simulink library "custom_lib"  (R2021a)
settings: Solver=VariableStepAuto  StartTime=0.0  StopTime=10.0  RelTol=1e-3
libraries: $bdroot x55
settings Model: Creator=Acer  LastModifiedBy=Acer

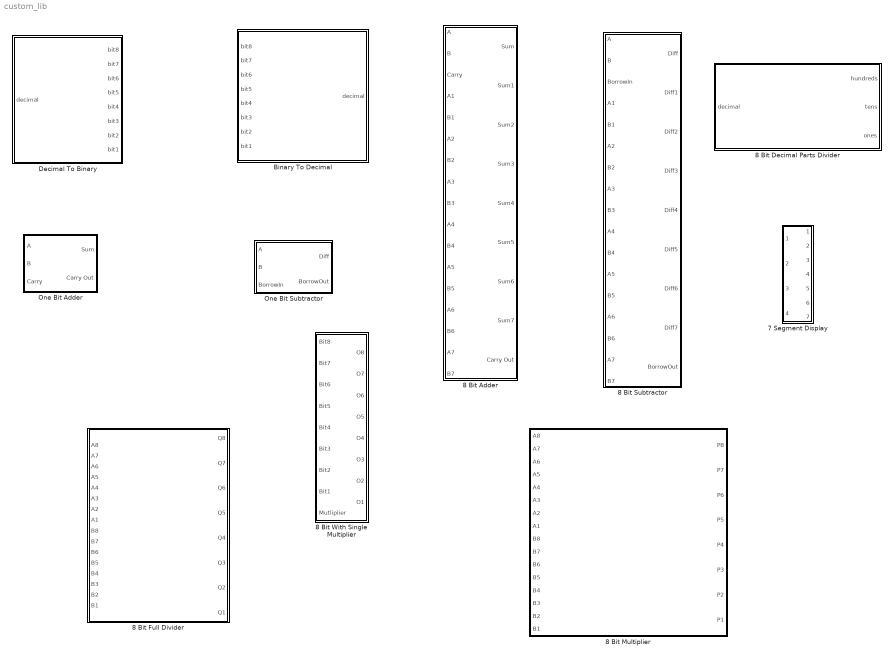
== system custom_lib ==
  7 Segment Display : Subsystem
  8 Bit Adder : Subsystem
  8 Bit Decimal Parts Divider : MATLAB Function  TreatAsAtomicUnit=on
  8 Bit Full Divider : Subsystem
  8 Bit Multiplier : Subsystem
  8 Bit Subtractor : Subsystem
  8 Bit With Single Multiplier : Subsystem
  Binary To Decimal : MATLAB Function  TreatAsAtomicUnit=on
  Decimal To Binary : MATLAB Function  TreatAsAtomicUnit=on
  One Bit Adder : Subsystem
  One Bit Subtractor : Subsystem

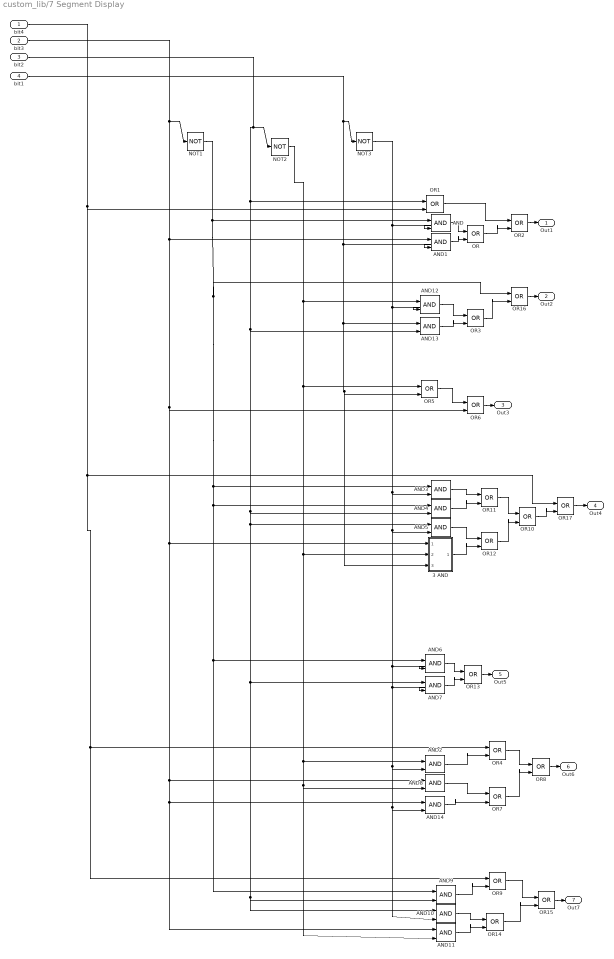
== system custom_lib/7 Segment Display ==
  bit4 : Inport
  bit3 : Inport  Port=2
  bit2 : Inport  Port=3
  bit1 : Inport  Port=4
  3 AND : Subsystem
  AND{,1..14} (15 alike) : Logic  IconShape=distinctive  AllPortsSameDT=off  OutDataTypeStr=boolean
  NOT1 : Logic  Operator=NOT  IconShape=distinctive  AllPortsSameDT=off  OutDataTypeStr=boolean
  NOT2 : Logic  Operator=NOT  IconShape=distinctive  AllPortsSameDT=off  OutDataTypeStr=boolean
  NOT3 : Logic  Operator=NOT  IconShape=distinctive  AllPortsSameDT=off  OutDataTypeStr=boolean
  OR{,1..17} (18 alike) : Logic  Operator=OR  IconShape=distinctive  AllPortsSameDT=off  OutDataTypeStr=boolean
  Out1 : Outport
  Out2 : Outport  Port=2
  Out3 : Outport  Port=3
  Out4 : Outport  Port=4
  Out5 : Outport  Port=5
  Out6 : Outport  Port=6
  Out7 : Outport  Port=7
  wires:
  OR16/1 -> Out2/1
  bit2/1 -> NOT2/1, OR1/1, AND13/2, AND5/1, AND10/1, AND9/2, AND7/1, AND4/2
  NOT2/1 -> OR5/1, AND2/1, AND11/2, AND8/2, 3 AND/2(In2), AND12/1
  bit3/1 -> NOT1/1, AND8/1, AND14/1, AND11/1, 3 AND/1(bit3), OR6/2, AND1/1
  AND7/1 -> OR13/2
  NOT3/1 -> AND/2, AND5/2, AND10/2, AND14/2, AND2/2, AND7/2, AND6/2, AND3/2, AND12/2
  NOT1/1 -> AND/1, OR16/1, AND4/1, AND9/1, AND6/1, AND3/1
  AND9/1 -> OR9/2
  OR3/1 -> OR16/2
  bit4/1 -> OR1/2, OR17/1, OR4/1, OR9/1
  OR4/1 -> OR8/1
  OR7/1 -> OR8/2
  OR17/1 -> Out4/1
  bit1/1 -> AND13/1, 3 AND/3(bit1), OR5/2, AND1/2, NOT3/1
  AND6/1 -> OR13/1
  AND10/1 -> OR14/1
  OR5/1 -> OR6/1
  OR14/1 -> OR15/2
  OR15/1 -> Out7/1
  OR9/1 -> OR15/1
  OR8/1 -> Out6/1
  OR/1 -> OR2/2
  AND2/1 -> OR4/2
  OR13/1 -> Out5/1
  AND8/1 -> OR7/1
  AND11/1 -> OR14/2
  AND12/1 -> OR3/1
  AND14/1 -> OR7/2
  OR1/1 -> OR2/1
  AND/1 -> OR/1
  AND1/1 -> OR/2
  AND13/1 -> OR3/2
  OR6/1 -> Out3/1
  OR2/1 -> Out1/1
  AND3/1 -> OR11/1
  AND4/1 -> OR11/2
  3 AND/1(Out1) -> OR12/2
  AND5/1 -> OR12/1
  OR11/1 -> OR10/1
  OR12/1 -> OR10/2
  OR10/1 -> OR17/2

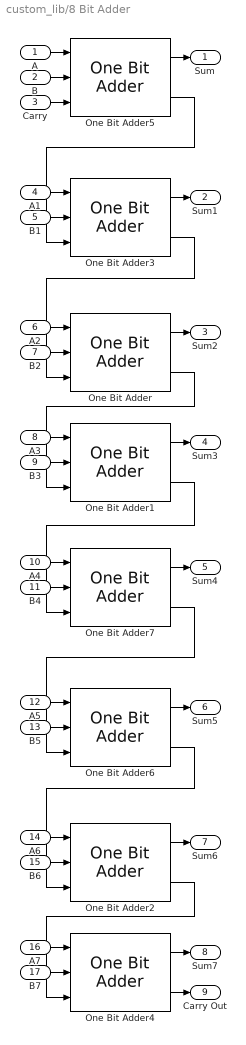
== system custom_lib/8 Bit Adder ==
  A : Inport
  B : Inport  Port=2
  Carry : Inport  Port=3
  A1 : Inport  Port=4
  B1 : Inport  Port=5
  A2 : Inport  Port=6
  B2 : Inport  Port=7
  A3 : Inport  Port=8
  B3 : Inport  Port=9
  A4 : Inport  Port=10
  B4 : Inport  Port=11
  A5 : Inport  Port=12
  B5 : Inport  Port=13
  A6 : Inport  Port=14
  B6 : Inport  Port=15
  A7 : Inport  Port=16
  B7 : Inport  Port=17
  One Bit Adder{,1..7} (8 alike) : $bdroot/One Bit Adder  SystemSampleTime=-1  VariantActivationTime=update diagram  Latency=0  AutoFrameSizeCalculation=off
  Sum : Outport
  Sum1 : Outport  Port=2
  Sum2 : Outport  Port=3
  Sum3 : Outport  Port=4
  Sum4 : Outport  Port=5
  Sum5 : Outport  Port=6
  Sum6 : Outport  Port=7
  Sum7 : Outport  Port=8
  Carry Out : Outport  Port=9
  wires:
  One Bit Adder2/1 -> Sum6/1
  One Bit Adder6/2 -> One Bit Adder2/3
  A1/1 -> One Bit Adder3/1
  One Bit Adder5/2 -> One Bit Adder3/3
  One Bit Adder3/1 -> Sum1/1
  A3/1 -> One Bit Adder1/1
  One Bit Adder7/2 -> One Bit Adder6/3
  One Bit Adder4/2 -> Carry Out/1
  One Bit Adder2/2 -> One Bit Adder4/3
  One Bit Adder3/2 -> One Bit Adder/3
  One Bit Adder/2 -> One Bit Adder1/3
  One Bit Adder1/2 -> One Bit Adder7/3
  One Bit Adder4/1 -> Sum7/1
  One Bit Adder1/1 -> Sum3/1
  B7/1 -> One Bit Adder4/2
  B5/1 -> One Bit Adder6/2
  B/1 -> One Bit Adder5/2
  B2/1 -> One Bit Adder/2
  B6/1 -> One Bit Adder2/2
  A4/1 -> One Bit Adder7/1
  B3/1 -> One Bit Adder1/2
  A2/1 -> One Bit Adder/1
  One Bit Adder/1 -> Sum2/1
  B1/1 -> One Bit Adder3/2
  A6/1 -> One Bit Adder2/1
  A5/1 -> One Bit Adder6/1
  One Bit Adder7/1 -> Sum4/1
  One Bit Adder5/1 -> Sum/1
  One Bit Adder6/1 -> Sum5/1
  B4/1 -> One Bit Adder7/2
  A7/1 -> One Bit Adder4/1
  A/1 -> One Bit Adder5/1
  Carry/1 -> One Bit Adder5/3

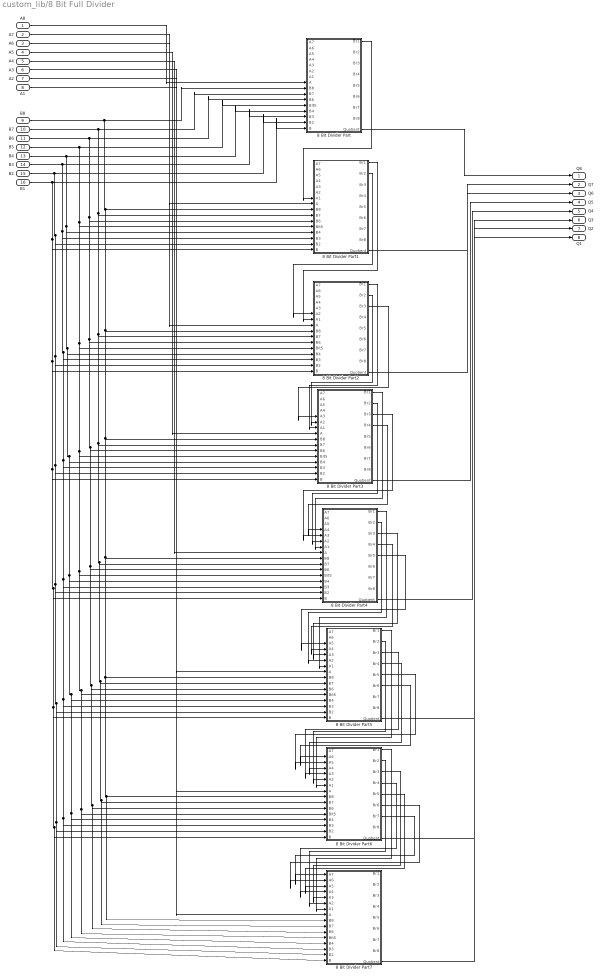
== system custom_lib/8 Bit Full Divider ==
  A8 : Inport
  A7 : Inport  Port=2
  A6 : Inport  Port=3
  A5 : Inport  Port=4
  A4 : Inport  Port=5
  A3 : Inport  Port=6
  A2 : Inport  Port=7
  A1 : Inport  Port=8
  B8 : Inport  Port=9
  B7 : Inport  Port=10
  B6 : Inport  Port=11
  B5 : Inport  Port=12
  B4 : Inport  Port=13
  B3 : Inport  Port=14
  B2 : Inport  Port=15
  B1 : Inport  Port=16
  8 Bit Divider Part : Subsystem
  8 Bit Divider Part1 : Subsystem
  8 Bit Divider Part2 : Subsystem
  8 Bit Divider Part3 : Subsystem
  8 Bit Divider Part4 : Subsystem
  8 Bit Divider Part5 : Subsystem
  8 Bit Divider Part6 : Subsystem
  8 Bit Divider Part7 : Subsystem
  Q8 : Outport
  Q7 : Outport  Port=2
  Q6 : Outport  Port=3
  Q5 : Outport  Port=4
  Q4 : Outport  Port=5
  Q3 : Outport  Port=6
  Q2 : Outport  Port=7
  Q1 : Outport  Port=8
  wires:
  B3/1 -> 8 Bit Divider Part7/14(B3), 8 Bit Divider Part6/14(B3), 8 Bit Divider Part5/14(B3), 8 Bit Divider Part4/14(B3), 8 Bit Divider Part3/14(B3), 8 Bit Divider Part2/14(B3), 8 Bit Divider Part1/14(B3), 8 Bit Divider Part/14(B3)
  B4/1 -> 8 Bit Divider Part7/13(B4), 8 Bit Divider Part6/13(B4), 8 Bit Divider Part5/13(B4), 8 Bit Divider Part4/13(B4), 8 Bit Divider Part3/13(B4), 8 Bit Divider Part2/13(B4), 8 Bit Divider Part1/13(B4), 8 Bit Divider Part/13(B4)
  8 Bit Divider Part2/1(Br1) -> 8 Bit Divider Part3/7(A1)
  8 Bit Divider Part4/1(Br1) -> 8 Bit Divider Part5/7(A1)
  B1/1 -> 8 Bit Divider Part7/16(B), 8 Bit Divider Part6/16(B), 8 Bit Divider Part5/16(B), 8 Bit Divider Part4/16(B), 8 Bit Divider Part3/16(B), 8 Bit Divider Part2/16(B), 8 Bit Divider Part1/16(B), 8 Bit Divider Part/16(B)
  8 Bit Divider Part4/5(Br5) -> 8 Bit Divider Part5/3(A5)
  8 Bit Divider Part6/5(Br5) -> 8 Bit Divider Part7/3(A5)
  A8/1 -> 8 Bit Divider Part/8(A)
  8 Bit Divider Part3/4(Br4) -> 8 Bit Divider Part4/4(A4)
  B2/1 -> 8 Bit Divider Part7/15(B2), 8 Bit Divider Part6/15(B2), 8 Bit Divider Part5/15(B2), 8 Bit Divider Part4/15(B2), 8 Bit Divider Part3/15(B2), 8 Bit Divider Part2/15(B2), 8 Bit Divider Part1/15(B2), 8 Bit Divider Part/15(B2)
  B8/1 -> 8 Bit Divider Part7/9(B8), 8 Bit Divider Part6/9(B8), 8 Bit Divider Part5/9(B8), 8 Bit Divider Part4/9(B8), 8 Bit Divider Part3/9(B8), 8 Bit Divider Part2/9(B8), 8 Bit Divider Part1/9(B8), 8 Bit Divider Part/9(B8)
  B7/1 -> 8 Bit Divider Part7/10(B7), 8 Bit Divider Part6/10(B7), 8 Bit Divider Part5/10(B7), 8 Bit Divider Part4/10(B7), 8 Bit Divider Part3/10(B7), 8 Bit Divider Part2/10(B7), 8 Bit Divider Part1/10(B7), 8 Bit Divider Part/10(B7)
  B6/1 -> 8 Bit Divider Part7/11(B6), 8 Bit Divider Part6/11(B6), 8 Bit Divider Part5/11(B6), 8 Bit Divider Part4/11(B6), 8 Bit Divider Part3/11(B6), 8 Bit Divider Part2/11(B6), 8 Bit Divider Part1/11(B6), 8 Bit Divider Part/11(B6)
  8 Bit Divider Part6/1(Br1) -> 8 Bit Divider Part7/7(A1)
  8 Bit Divider Part2/3(Br3) -> 8 Bit Divider Part3/5(A3)
  8 Bit Divider Part4/2(Br2) -> 8 Bit Divider Part5/6(A2)
  B5/1 -> 8 Bit Divider Part7/12(Bit5), 8 Bit Divider Part6/12(Bit5), 8 Bit Divider Part5/12(Bit5), 8 Bit Divider Part4/12(Bit5), 8 Bit Divider Part3/12(Bit5), 8 Bit Divider Part2/12(Bit5), 8 Bit Divider Part1/12(Bit5), 8 Bit Divider Part/12(Bit5)
  8 Bit Divider Part5/3(Br3) -> 8 Bit Divider Part6/5(A3)
  8 Bit Divider Part3/3(Br3) -> 8 Bit Divider Part4/5(A3)
  8 Bit Divider Part4/3(Br3) -> 8 Bit Divider Part5/5(A3)
  8 Bit Divider Part3/1(Br1) -> 8 Bit Divider Part4/7(A1)
  8 Bit Divider Part5/1(Br1) -> 8 Bit Divider Part6/7(A1)
  8 Bit Divider Part1/1(Br1) -> 8 Bit Divider Part2/7(A1)
  8 Bit Divider Part/1(Br1) -> 8 Bit Divider Part1/7(A1)
  8 Bit Divider Part1/2(Br2) -> 8 Bit Divider Part2/6(A2)
  8 Bit Divider Part6/2(Br2) -> 8 Bit Divider Part7/6(A2)
  A2/1 -> 8 Bit Divider Part6/8(A)
  8 Bit Divider Part2/2(Br2) -> 8 Bit Divider Part3/6(A2)
  8 Bit Divider Part6/4(Br4) -> 8 Bit Divider Part7/4(A4)
  8 Bit Divider Part6/3(Br3) -> 8 Bit Divider Part7/5(A3)
  8 Bit Divider Part5/4(Br4) -> 8 Bit Divider Part6/4(A4)
  8 Bit Divider Part3/2(Br2) -> 8 Bit Divider Part4/6(A2)
  8 Bit Divider Part5/6(Br6) -> 8 Bit Divider Part6/2(A6)
  8 Bit Divider Part4/4(Br4) -> 8 Bit Divider Part5/4(A4)
  8 Bit Divider Part6/6(Br6) -> 8 Bit Divider Part7/2(A6)
  A5/1 -> 8 Bit Divider Part3/8(A)
  8 Bit Divider Part5/2(Br2) -> 8 Bit Divider Part6/6(A2)
  8 Bit Divider Part1/9(Quotient) -> Q7/1
  8 Bit Divider Part2/9(Quotient) -> Q6/1
  8 Bit Divider Part5/5(Br5) -> 8 Bit Divider Part6/3(A5)
  8 Bit Divider Part6/7(Br7) -> 8 Bit Divider Part7/1(A7)
  8 Bit Divider Part/9(Quotient) -> Q8/1
  A6/1 -> 8 Bit Divider Part2/8(A)
  A7/1 -> 8 Bit Divider Part1/8(A)
  A1/1 -> 8 Bit Divider Part7/8(A)
  A4/1 -> 8 Bit Divider Part4/8(A)
  8 Bit Divider Part6/9(Quotient) -> Q2/1
  8 Bit Divider Part5/9(Quotient) -> Q3/1
  A3/1 -> 8 Bit Divider Part5/8(A)
  8 Bit Divider Part3/9(Quotient) -> Q5/1
  8 Bit Divider Part4/9(Quotient) -> Q4/1
  8 Bit Divider Part7/9(Quotient) -> Q1/1

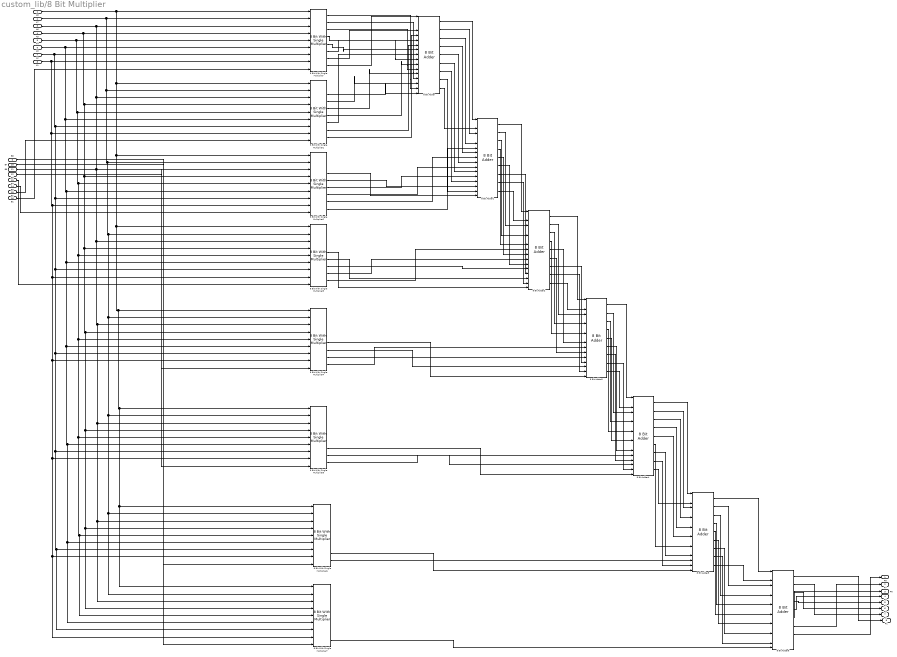
== system custom_lib/8 Bit Multiplier ==
  A8 : Inport
  A7 : Inport  Port=2
  A6 : Inport  Port=3
  A5 : Inport  Port=4
  A4 : Inport  Port=5
  A3 : Inport  Port=6
  A2 : Inport  Port=7
  A1 : Inport  Port=8
  B8 : Inport  Port=9
  B7 : Inport  Port=10
  B6 : Inport  Port=11
  B5 : Inport  Port=12
  B4 : Inport  Port=13
  B3 : Inport  Port=14
  B2 : Inport  Port=15
  B1 : Inport  Port=16
  8 Bit Adder{,1..6} (7 alike) : $bdroot/8 Bit Adder  SystemSampleTime=-1  VariantActivationTime=update diagram  Latency=0  AutoFrameSizeCalculation=off
  8 Bit With Single Multiplier{,1..7} (8 alike) : $bdroot/8 Bit With Single Multiplier  SystemSampleTime=-1  VariantActivationTime=update diagram  Latency=0  AutoFrameSizeCalculation=off
  P8 : Outport
  P7 : Outport  Port=2
  P6 : Outport  Port=3
  P5 : Outport  Port=4
  P4 : Outport  Port=5
  P3 : Outport  Port=6
  P2 : Outport  Port=7
  P1 : Outport  Port=8
  wires:
  8 Bit With Single Multiplier2/5 -> 8 Bit Adder1/13
  A5/1 -> 8 Bit With Single Multiplier7/4, 8 Bit With Single Multiplier6/4, 8 Bit With Single Multiplier5/4, 8 Bit With Single Multiplier4/4, 8 Bit With Single Multiplier3/4, 8 Bit With Single Multiplier2/4, 8 Bit With Single Multiplier1/4, 8 Bit With Single Multiplier/4
  A1/1 -> 8 Bit With Single Multiplier7/8, 8 Bit With Single Multiplier6/8, 8 Bit With Single Multiplier5/8, 8 Bit With Single Multiplier4/8, 8 Bit With Single Multiplier3/8, 8 Bit With Single Multiplier2/8, 8 Bit With Single Multiplier1/8, 8 Bit With Single Multiplier/8
  8 Bit With Single Multiplier3/4 -> 8 Bit Adder2/17
  8 Bit With Single Multiplier5/7 -> 8 Bit Adder4/15
  A2/1 -> 8 Bit With Single Multiplier7/7, 8 Bit With Single Multiplier6/7, 8 Bit With Single Multiplier5/7, 8 Bit With Single Multiplier4/7, 8 Bit With Single Multiplier3/7, 8 Bit With Single Multiplier2/7, 8 Bit With Single Multiplier1/7, 8 Bit With Single Multiplier/7
  8 Bit With Single Multiplier/1 -> 8 Bit Adder/16
  8 Bit With Single Multiplier/2 -> 8 Bit Adder/14
  8 Bit Adder5/2 -> 8 Bit Adder6/4
  8 Bit Adder6/5 -> P5/1
  8 Bit Adder1/4 -> 8 Bit Adder2/8
  8 Bit With Single Multiplier7/8 -> 8 Bit Adder6/17
  8 Bit With Single Multiplier5/6 -> 8 Bit Adder4/17
  8 Bit Adder4/3 -> 8 Bit Adder5/6
  8 Bit Adder3/2 -> 8 Bit Adder4/4
  8 Bit Adder4/2 -> 8 Bit Adder5/4
  8 Bit Adder/2 -> 8 Bit Adder1/4
  8 Bit With Single Multiplier/3 -> 8 Bit Adder/12
  8 Bit Adder5/1 -> 8 Bit Adder6/1
  8 Bit Adder2/4 -> 8 Bit Adder3/8
  8 Bit With Single Multiplier/4 -> 8 Bit Adder/10
  8 Bit Adder4/9 -> 8 Bit Adder5/3
  8 Bit Adder1/9 -> 8 Bit Adder2/3
  8 Bit Adder2/1 -> 8 Bit Adder3/1
  8 Bit With Single Multiplier3/5 -> 8 Bit Adder2/15
  8 Bit Adder5/7 -> 8 Bit Adder6/14
  A8/1 -> 8 Bit With Single Multiplier7/1, 8 Bit With Single Multiplier6/1, 8 Bit With Single Multiplier5/1, 8 Bit With Single Multiplier4/1, 8 Bit With Single Multiplier3/1, 8 Bit With Single Multiplier2/1, 8 Bit With Single Multiplier1/1, 8 Bit With Single Multiplier/1
  8 Bit Adder1/6 -> 8 Bit Adder2/12
  8 Bit Adder5/5 -> 8 Bit Adder6/10
  8 Bit With Single Multiplier2/4 -> 8 Bit Adder1/15
  8 Bit With Single Multiplier/8 -> 8 Bit Adder/1
  8 Bit With Single Multiplier2/7 -> 8 Bit Adder1/9
  8 Bit Adder6/3 -> P3/1
  8 Bit With Single Multiplier1/2 -> 8 Bit Adder/17
  A7/1 -> 8 Bit With Single Multiplier7/2, 8 Bit With Single Multiplier6/2, 8 Bit With Single Multiplier5/2, 8 Bit With Single Multiplier4/2, 8 Bit With Single Multiplier3/2, 8 Bit With Single Multiplier2/2, 8 Bit With Single Multiplier1/2, 8 Bit With Single Multiplier/2
  8 Bit Adder6/2 -> P2/1
  8 Bit With Single Multiplier1/4 -> 8 Bit Adder/13
  8 Bit Adder/1 -> 8 Bit Adder1/1
  A6/1 -> 8 Bit With Single Multiplier7/3, 8 Bit With Single Multiplier6/3, 8 Bit With Single Multiplier5/3, 8 Bit With Single Multiplier4/3, 8 Bit With Single Multiplier3/3, 8 Bit With Single Multiplier2/3, 8 Bit With Single Multiplier1/3, 8 Bit With Single Multiplier/3
  8 Bit Adder/6 -> 8 Bit Adder1/12
  8 Bit Adder1/7 -> 8 Bit Adder2/14
  8 Bit Adder/7 -> 8 Bit Adder1/14
  8 Bit Adder1/8 -> 8 Bit Adder2/16
  A3/1 -> 8 Bit With Single Multiplier7/6, 8 Bit With Single Multiplier6/6, 8 Bit With Single Multiplier5/6, 8 Bit With Single Multiplier4/6, 8 Bit With Single Multiplier3/6, 8 Bit With Single Multiplier2/6, 8 Bit With Single Multiplier1/6, 8 Bit With Single Multiplier/6
  8 Bit With Single Multiplier3/6 -> 8 Bit Adder2/13
  8 Bit With Single Multiplier1/7 -> 8 Bit Adder/7
  8 Bit With Single Multiplier2/8 -> 8 Bit Adder1/7
  8 Bit Adder/3 -> 8 Bit Adder1/6
  8 Bit Adder/5 -> 8 Bit Adder1/10
  8 Bit Adder3/1 -> 8 Bit Adder4/1
  8 Bit Adder1/3 -> 8 Bit Adder2/6
  8 Bit With Single Multiplier1/5 -> 8 Bit Adder/11
  B2/1 -> 8 Bit With Single Multiplier1/9
  8 Bit Adder1/2 -> 8 Bit Adder2/4
  8 Bit Adder/4 -> 8 Bit Adder1/8
  B3/1 -> 8 Bit With Single Multiplier2/9
  8 Bit Adder5/6 -> 8 Bit Adder6/12
  8 Bit Adder1/1 -> 8 Bit Adder2/1
  A4/1 -> 8 Bit With Single Multiplier7/5, 8 Bit With Single Multiplier6/5, 8 Bit With Single Multiplier5/5, 8 Bit With Single Multiplier4/5, 8 Bit With Single Multiplier3/5, 8 Bit With Single Multiplier2/5, 8 Bit With Single Multiplier1/5, 8 Bit With Single Multiplier/5
  8 Bit Adder2/6 -> 8 Bit Adder3/12
  8 Bit Adder2/9 -> 8 Bit Adder3/3
  8 Bit With Single Multiplier1/6 -> 8 Bit Adder/9
  8 Bit Adder3/6 -> 8 Bit Adder4/12
  8 Bit With Single Multiplier/6 -> 8 Bit Adder/6
  8 Bit Adder3/7 -> 8 Bit Adder4/14
  8 Bit Adder2/3 -> 8 Bit Adder3/6
  8 Bit Adder2/5 -> 8 Bit Adder3/10
  8 Bit With Single Multiplier5/8 -> 8 Bit Adder4/13
  8 Bit Adder1/5 -> 8 Bit Adder2/10
  8 Bit Adder2/8 -> 8 Bit Adder3/16
  8 Bit With Single Multiplier3/8 -> 8 Bit Adder2/9
  8 Bit With Single Multiplier4/7 -> 8 Bit Adder3/13
  8 Bit With Single Multiplier/5 -> 8 Bit Adder/8
  8 Bit With Single Multiplier1/3 -> 8 Bit Adder/15
  8 Bit Adder6/4 -> P4/1
  8 Bit Adder3/3 -> 8 Bit Adder4/6
  8 Bit With Single Multiplier4/6 -> 8 Bit Adder3/15
  8 Bit Adder3/9 -> 8 Bit Adder4/3
  8 Bit With Single Multiplier/7 -> 8 Bit Adder/4
  8 Bit Adder3/4 -> 8 Bit Adder4/8
  8 Bit With Single Multiplier6/7 -> 8 Bit Adder5/17
  8 Bit Adder4/4 -> 8 Bit Adder5/8
  8 Bit Adder2/7 -> 8 Bit Adder3/14
  8 Bit With Single Multiplier1/8 -> 8 Bit Adder/5
  8 Bit With Single Multiplier6/8 -> 8 Bit Adder5/15
  8 Bit Adder4/5 -> 8 Bit Adder5/10
  8 Bit With Single Multiplier2/6 -> 8 Bit Adder1/11
  8 Bit Adder4/6 -> 8 Bit Adder5/12
  8 Bit Adder4/1 -> 8 Bit Adder5/1
  8 Bit Adder3/5 -> 8 Bit Adder4/10
  8 Bit Adder2/2 -> 8 Bit Adder3/4
  8 Bit Adder3/8 -> 8 Bit Adder4/16
  8 Bit Adder/8 -> 8 Bit Adder1/16
  8 Bit Adder5/3 -> 8 Bit Adder6/6
  8 Bit Adder5/4 -> 8 Bit Adder6/8
  8 Bit Adder4/8 -> 8 Bit Adder5/16
  8 Bit Adder5/8 -> 8 Bit Adder6/16
  8 Bit With Single Multiplier2/3 -> 8 Bit Adder1/17
  8 Bit Adder4/7 -> 8 Bit Adder5/14
  8 Bit Adder5/9 -> 8 Bit Adder6/3
  8 Bit With Single Multiplier4/5 -> 8 Bit Adder3/17
  8 Bit With Single Multiplier4/8 -> 8 Bit Adder3/11
  8 Bit Adder/9 -> 8 Bit Adder1/3
  8 Bit With Single Multiplier3/7 -> 8 Bit Adder2/11
  8 Bit Adder6/6 -> P6/1
  B5/1 -> 8 Bit With Single Multiplier4/9
  B7/1 -> 8 Bit With Single Multiplier6/9
  B4/1 -> 8 Bit With Single Multiplier3/9
  B8/1 -> 8 Bit With Single Multiplier7/9
  8 Bit Adder6/8 -> P8/1
  B6/1 -> 8 Bit With Single Multiplier5/9
  B1/1 -> 8 Bit With Single Multiplier/9
  8 Bit Adder6/1 -> P1/1
  8 Bit Adder6/7 -> P7/1

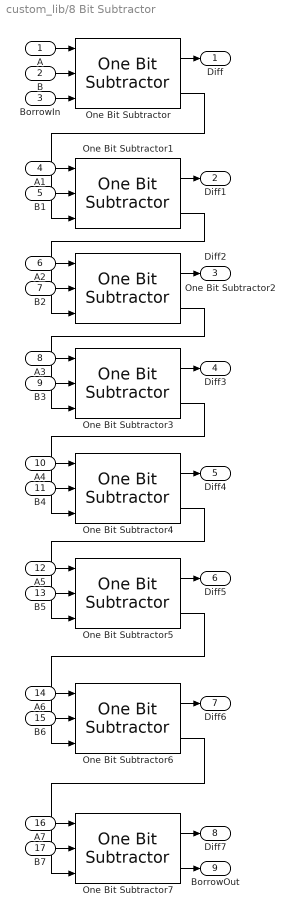
== system custom_lib/8 Bit Subtractor ==
  A : Inport
  B : Inport  Port=2
  BorrowIn : Inport  Port=3
  A1 : Inport  Port=4
  B1 : Inport  Port=5
  A2 : Inport  Port=6
  B2 : Inport  Port=7
  A3 : Inport  Port=8
  B3 : Inport  Port=9
  A4 : Inport  Port=10
  B4 : Inport  Port=11
  A5 : Inport  Port=12
  B5 : Inport  Port=13
  A6 : Inport  Port=14
  B6 : Inport  Port=15
  A7 : Inport  Port=16
  B7 : Inport  Port=17
  One Bit Subtractor{,1..7} (8 alike) : $bdroot/One Bit Subtractor  SystemSampleTime=-1  VariantActivationTime=update diagram  Latency=0  AutoFrameSizeCalculation=off
  Diff : Outport
  Diff1 : Outport  Port=2
  Diff2 : Outport  Port=3
  Diff3 : Outport  Port=4
  Diff4 : Outport  Port=5
  Diff5 : Outport  Port=6
  Diff6 : Outport  Port=7
  Diff7 : Outport  Port=8
  BorrowOut : Outport  Port=9
  wires:
  One Bit Subtractor1/2 -> One Bit Subtractor2/3
  B2/1 -> One Bit Subtractor2/2
  One Bit Subtractor2/2 -> One Bit Subtractor3/3
  One Bit Subtractor3/2 -> One Bit Subtractor4/3
  A3/1 -> One Bit Subtractor3/1
  One Bit Subtractor5/2 -> One Bit Subtractor6/3
  One Bit Subtractor/2 -> One Bit Subtractor1/3
  One Bit Subtractor6/2 -> One Bit Subtractor7/3
  B5/1 -> One Bit Subtractor5/2
  One Bit Subtractor4/2 -> One Bit Subtractor5/3
  B1/1 -> One Bit Subtractor1/2
  One Bit Subtractor5/1 -> Diff5/1
  B6/1 -> One Bit Subtractor6/2
  One Bit Subtractor6/1 -> Diff6/1
  BorrowIn/1 -> One Bit Subtractor/3
  One Bit Subtractor3/1 -> Diff3/1
  One Bit Subtractor4/1 -> Diff4/1
  A5/1 -> One Bit Subtractor5/1
  A2/1 -> One Bit Subtractor2/1
  One Bit Subtractor2/1 -> Diff2/1
  B4/1 -> One Bit Subtractor4/2
  A6/1 -> One Bit Subtractor6/1
  A4/1 -> One Bit Subtractor4/1
  One Bit Subtractor7/1 -> Diff7/1
  B/1 -> One Bit Subtractor/2
  One Bit Subtractor1/1 -> Diff1/1
  A7/1 -> One Bit Subtractor7/1
  A1/1 -> One Bit Subtractor1/1
  A/1 -> One Bit Subtractor/1
  One Bit Subtractor/1 -> Diff/1
  B3/1 -> One Bit Subtractor3/2
  B7/1 -> One Bit Subtractor7/2
  One Bit Subtractor7/2 -> BorrowOut/1

== system custom_lib/8 Bit With Single Multiplier ==
  Bit8 : Inport
  Bit7 : Inport  Port=2
  Bit6 : Inport  Port=3
  Bit5 : Inport  Port=4
  Bit4 : Inport  Port=5
  Bit3 : Inport  Port=6
  Bit2 : Inport  Port=7
  Bit1 : Inport  Port=8
  Mutliplier : Inport  Port=9
  AND{,1..7} (8 alike) : Logic  IconShape=distinctive  AllPortsSameDT=off  OutDataTypeStr=boolean
  O8 : Outport
  O7 : Outport  Port=2
  O6 : Outport  Port=3
  O5 : Outport  Port=4
  O4 : Outport  Port=5
  O3 : Outport  Port=6
  O2 : Outport  Port=7
  O1 : Outport  Port=8
  wires:
  Mutliplier/1 -> AND/2, AND1/2, AND2/2, AND3/2, AND6/2, AND7/2, AND5/2, AND4/2
  AND/1 -> O8/1
  AND3/1 -> O5/1
  Bit8/1 -> AND/1
  Bit5/1 -> AND3/1
  AND2/1 -> O6/1
  AND5/1 -> O2/1
  AND7/1 -> O3/1
  Bit3/1 -> AND7/1
  Bit1/1 -> AND4/1
  Bit4/1 -> AND6/1
  AND6/1 -> O4/1
  Bit7/1 -> AND1/1
  Bit2/1 -> AND5/1
  AND1/1 -> O7/1
  Bit6/1 -> AND2/1
  AND4/1 -> O1/1

== system custom_lib/One Bit Adder ==
  A : Inport
  B : Inport  Port=2
  Carry : Inport  Port=3
  AND : Logic  IconShape=distinctive  AllPortsSameDT=off  OutDataTypeStr=boolean
  AND1 : Logic  IconShape=distinctive  AllPortsSameDT=off  OutDataTypeStr=boolean
  OR : Logic  Operator=OR  IconShape=distinctive  AllPortsSameDT=off  OutDataTypeStr=boolean
  XOR : Logic  Operator=XOR  IconShape=distinctive  AllPortsSameDT=off  OutDataTypeStr=boolean
  XOR1 : Logic  Operator=XOR  IconShape=distinctive  AllPortsSameDT=off  OutDataTypeStr=boolean
  Sum : Outport
  Carry Out : Outport  Port=2
  wires:
  AND1/1 -> OR/2
  XOR1/1 -> Sum/1
  Carry/1 -> XOR1/2, AND/2
  B/1 -> AND1/2, XOR/2
  A/1 -> AND1/1, XOR/1
  OR/1 -> Carry Out/1
  AND/1 -> OR/1
  XOR/1 -> AND/1, XOR1/1

== system custom_lib/One Bit Subtractor ==
  A : Inport
  B : Inport  Port=2
  BorrowIn : Inport  Port=3
  AND : Logic  IconShape=distinctive  AllPortsSameDT=off  OutDataTypeStr=boolean
  AND1 : Logic  IconShape=distinctive  AllPortsSameDT=off  OutDataTypeStr=boolean
  NOT : Logic  Operator=NOT  IconShape=distinctive  AllPortsSameDT=off  OutDataTypeStr=boolean
  NOT1 : Logic  Operator=NOT  IconShape=distinctive  AllPortsSameDT=off  OutDataTypeStr=boolean
  OR : Logic  Operator=OR  IconShape=distinctive  AllPortsSameDT=off  OutDataTypeStr=boolean
  XOR : Logic  Operator=XOR  IconShape=distinctive  AllPortsSameDT=off  OutDataTypeStr=boolean
  XOR1 : Logic  Operator=XOR  IconShape=distinctive  AllPortsSameDT=off  OutDataTypeStr=boolean
  Diff : Outport
  BorrowOut : Outport  Port=2
  wires:
  BorrowIn/1 -> AND1/2, XOR1/2
  AND/1 -> OR/2
  A/1 -> NOT/1, XOR/1
  B/1 -> AND/2, XOR/2
  XOR/1 -> NOT1/1, XOR1/1
  NOT1/1 -> AND1/1
  XOR1/1 -> Diff/1
  NOT/1 -> AND/1
  AND1/1 -> OR/1
  OR/1 -> BorrowOut/1

== system custom_lib/7 Segment Display/3 AND ==
  bit3 : Inport
  In2 : Inport  Port=2
  bit1 : Inport  Port=3
  AND15 : Logic  IconShape=distinctive  AllPortsSameDT=off  OutDataTypeStr=boolean
  AND16 : Logic  IconShape=distinctive  AllPortsSameDT=off  OutDataTypeStr=boolean
  Out1 : Outport
  wires:
  In2/1 -> AND15/2
  AND16/1 -> Out1/1
  AND15/1 -> AND16/1
  bit3/1 -> AND15/1
  bit1/1 -> AND16/2

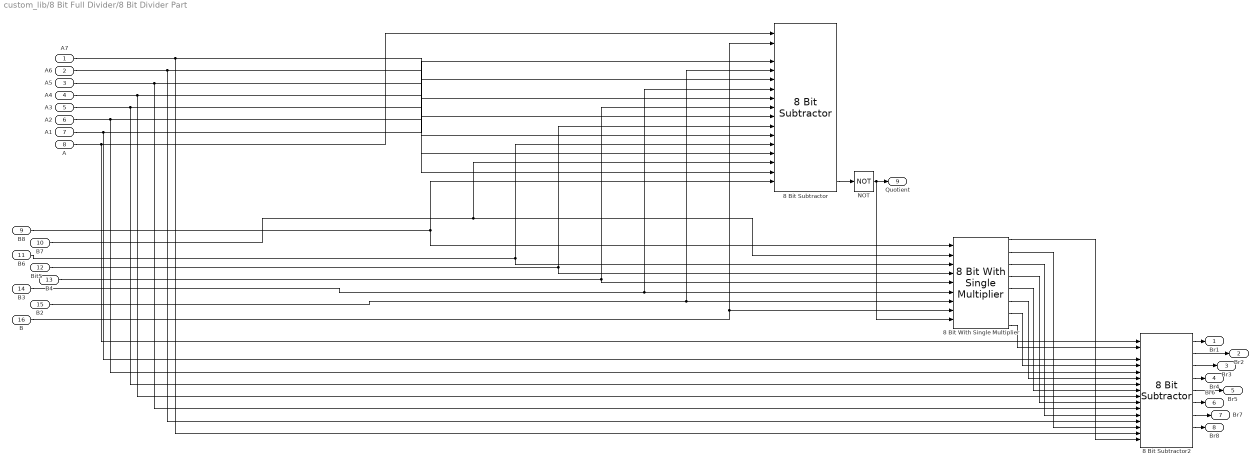
== system custom_lib/8 Bit Full Divider/8 Bit Divider Part ==
  A7 : Inport
  A6 : Inport  Port=2
  A5 : Inport  Port=3
  A4 : Inport  Port=4
  A3 : Inport  Port=5
  A2 : Inport  Port=6
  A1 : Inport  Port=7
  A : Inport  Port=8
  B8 : Inport  Port=9
  B7 : Inport  Port=10
  B6 : Inport  Port=11
  Bit5 : Inport  Port=12
  B4 : Inport  Port=13
  B3 : Inport  Port=14
  B2 : Inport  Port=15
  B : Inport  Port=16
  8 Bit Subtractor : $bdroot/8 Bit Subtractor  SystemSampleTime=-1  VariantActivationTime=update diagram  Latency=0  AutoFrameSizeCalculation=off
  8 Bit Subtractor2 : $bdroot/8 Bit Subtractor  SystemSampleTime=-1  VariantActivationTime=update diagram  Latency=0  AutoFrameSizeCalculation=off
  8 Bit With Single Multiplier : $bdroot/8 Bit With Single Multiplier  SystemSampleTime=-1  VariantActivationTime=update diagram  Latency=0  AutoFrameSizeCalculation=off
  NOT : Logic  Operator=NOT  IconShape=distinctive  AllPortsSameDT=off  OutDataTypeStr=boolean
  Br1 : Outport
  Br2 : Outport  Port=2
  Br3 : Outport  Port=3
  Br4 : Outport  Port=4
  Br5 : Outport  Port=5
  Br6 : Outport  Port=6
  Br7 : Outport  Port=7
  Br8 : Outport  Port=8
  Quotient : Outport  Port=9
  wires:
  8 Bit Subtractor2/3 -> Br3/1
  8 Bit With Single Multiplier/2 -> 8 Bit Subtractor2/15
  8 Bit With Single Multiplier/7 -> 8 Bit Subtractor2/5
  B2/1 -> 8 Bit Subtractor/5, 8 Bit With Single Multiplier/7
  B6/1 -> 8 Bit Subtractor/13, 8 Bit With Single Multiplier/3
  8 Bit With Single Multiplier/1 -> 8 Bit Subtractor2/17
  8 Bit Subtractor2/6 -> Br6/1
  A7/1 -> 8 Bit Subtractor2/16, 8 Bit Subtractor/16
  NOT/1 -> Quotient/1, 8 Bit With Single Multiplier/9
  B8/1 -> 8 Bit Subtractor/17, 8 Bit With Single Multiplier/1
  A/1 -> 8 Bit Subtractor2/1, 8 Bit Subtractor/1
  A3/1 -> 8 Bit Subtractor2/8, 8 Bit Subtractor/8
  8 Bit Subtractor2/8 -> Br8/1
  B4/1 -> 8 Bit Subtractor/9, 8 Bit With Single Multiplier/5
  A2/1 -> 8 Bit Subtractor2/6, 8 Bit Subtractor/6
  8 Bit Subtractor2/2 -> Br2/1
  8 Bit With Single Multiplier/3 -> 8 Bit Subtractor2/13
  B7/1 -> 8 Bit With Single Multiplier/2, 8 Bit Subtractor/15
  8 Bit Subtractor/9 -> NOT/1
  B3/1 -> 8 Bit Subtractor/7, 8 Bit With Single Multiplier/6
  Bit5/1 -> 8 Bit Subtractor/11, 8 Bit With Single Multiplier/4
  8 Bit With Single Multiplier/8 -> 8 Bit Subtractor2/2
  8 Bit With Single Multiplier/5 -> 8 Bit Subtractor2/9
  8 Bit With Single Multiplier/6 -> 8 Bit Subtractor2/7
  8 Bit Subtractor2/4 -> Br4/1
  8 Bit Subtractor2/7 -> Br7/1
  8 Bit With Single Multiplier/4 -> 8 Bit Subtractor2/11
  B/1 -> 8 Bit With Single Multiplier/8, 8 Bit Subtractor/2
  8 Bit Subtractor2/5 -> Br5/1
  A1/1 -> 8 Bit Subtractor2/4, 8 Bit Subtractor/4
  A6/1 -> 8 Bit Subtractor2/14, 8 Bit Subtractor/14
  8 Bit Subtractor2/1 -> Br1/1
  A4/1 -> 8 Bit Subtractor2/10, 8 Bit Subtractor/10
  A5/1 -> 8 Bit Subtractor2/12, 8 Bit Subtractor/12

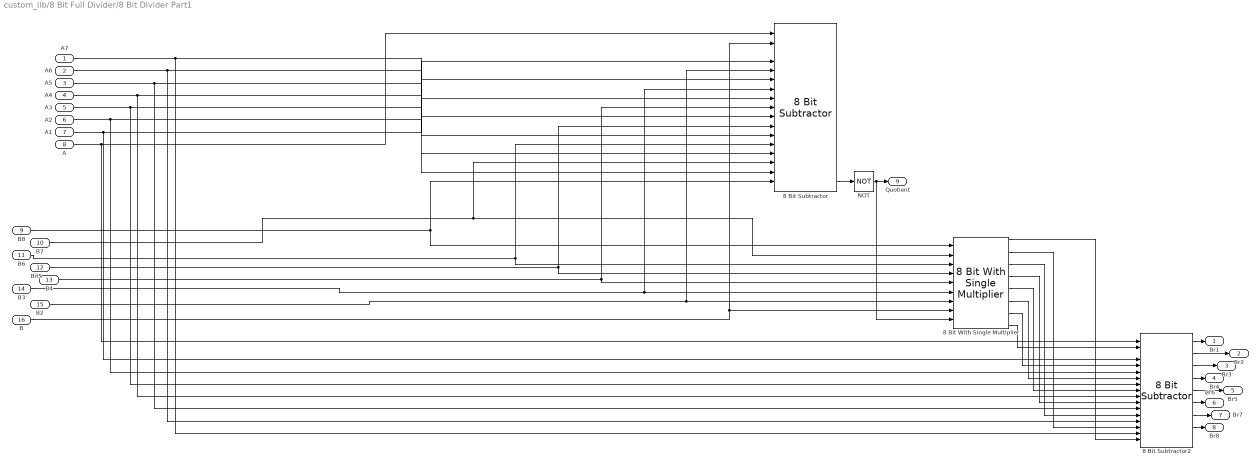
== system custom_lib/8 Bit Full Divider/8 Bit Divider Part1 ==
  A7 : Inport
  A6 : Inport  Port=2
  A5 : Inport  Port=3
  A4 : Inport  Port=4
  A3 : Inport  Port=5
  A2 : Inport  Port=6
  A1 : Inport  Port=7
  A : Inport  Port=8
  B8 : Inport  Port=9
  B7 : Inport  Port=10
  B6 : Inport  Port=11
  Bit5 : Inport  Port=12
  B4 : Inport  Port=13
  B3 : Inport  Port=14
  B2 : Inport  Port=15
  B : Inport  Port=16
  8 Bit Subtractor : $bdroot/8 Bit Subtractor  SystemSampleTime=-1  VariantActivationTime=update diagram  Latency=0  AutoFrameSizeCalculation=off
  8 Bit Subtractor2 : $bdroot/8 Bit Subtractor  SystemSampleTime=-1  VariantActivationTime=update diagram  Latency=0  AutoFrameSizeCalculation=off
  8 Bit With Single Multiplier : $bdroot/8 Bit With Single Multiplier  SystemSampleTime=-1  VariantActivationTime=update diagram  Latency=0  AutoFrameSizeCalculation=off
  NOT : Logic  Operator=NOT  IconShape=distinctive  AllPortsSameDT=off  OutDataTypeStr=boolean
  Br1 : Outport
  Br2 : Outport  Port=2
  Br3 : Outport  Port=3
  Br4 : Outport  Port=4
  Br5 : Outport  Port=5
  Br6 : Outport  Port=6
  Br7 : Outport  Port=7
  Br8 : Outport  Port=8
  Quotient : Outport  Port=9
  wires:
  8 Bit Subtractor2/3 -> Br3/1
  8 Bit With Single Multiplier/2 -> 8 Bit Subtractor2/15
  8 Bit With Single Multiplier/7 -> 8 Bit Subtractor2/5
  B2/1 -> 8 Bit Subtractor/5, 8 Bit With Single Multiplier/7
  B6/1 -> 8 Bit Subtractor/13, 8 Bit With Single Multiplier/3
  8 Bit With Single Multiplier/1 -> 8 Bit Subtractor2/17
  8 Bit Subtractor2/6 -> Br6/1
  A7/1 -> 8 Bit Subtractor2/16, 8 Bit Subtractor/16
  NOT/1 -> Quotient/1, 8 Bit With Single Multiplier/9
  B8/1 -> 8 Bit Subtractor/17, 8 Bit With Single Multiplier/1
  A/1 -> 8 Bit Subtractor2/1, 8 Bit Subtractor/1
  A3/1 -> 8 Bit Subtractor2/8, 8 Bit Subtractor/8
  8 Bit Subtractor2/8 -> Br8/1
  B4/1 -> 8 Bit Subtractor/9, 8 Bit With Single Multiplier/5
  A2/1 -> 8 Bit Subtractor2/6, 8 Bit Subtractor/6
  8 Bit Subtractor2/2 -> Br2/1
  8 Bit With Single Multiplier/3 -> 8 Bit Subtractor2/13
  B7/1 -> 8 Bit With Single Multiplier/2, 8 Bit Subtractor/15
  8 Bit Subtractor/9 -> NOT/1
  B3/1 -> 8 Bit Subtractor/7, 8 Bit With Single Multiplier/6
  Bit5/1 -> 8 Bit Subtractor/11, 8 Bit With Single Multiplier/4
  8 Bit With Single Multiplier/8 -> 8 Bit Subtractor2/2
  8 Bit With Single Multiplier/5 -> 8 Bit Subtractor2/9
  8 Bit With Single Multiplier/6 -> 8 Bit Subtractor2/7
  8 Bit Subtractor2/4 -> Br4/1
  8 Bit Subtractor2/7 -> Br7/1
  8 Bit With Single Multiplier/4 -> 8 Bit Subtractor2/11
  B/1 -> 8 Bit With Single Multiplier/8, 8 Bit Subtractor/2
  8 Bit Subtractor2/5 -> Br5/1
  A1/1 -> 8 Bit Subtractor2/4, 8 Bit Subtractor/4
  A6/1 -> 8 Bit Subtractor2/14, 8 Bit Subtractor/14
  8 Bit Subtractor2/1 -> Br1/1
  A4/1 -> 8 Bit Subtractor2/10, 8 Bit Subtractor/10
  A5/1 -> 8 Bit Subtractor2/12, 8 Bit Subtractor/12

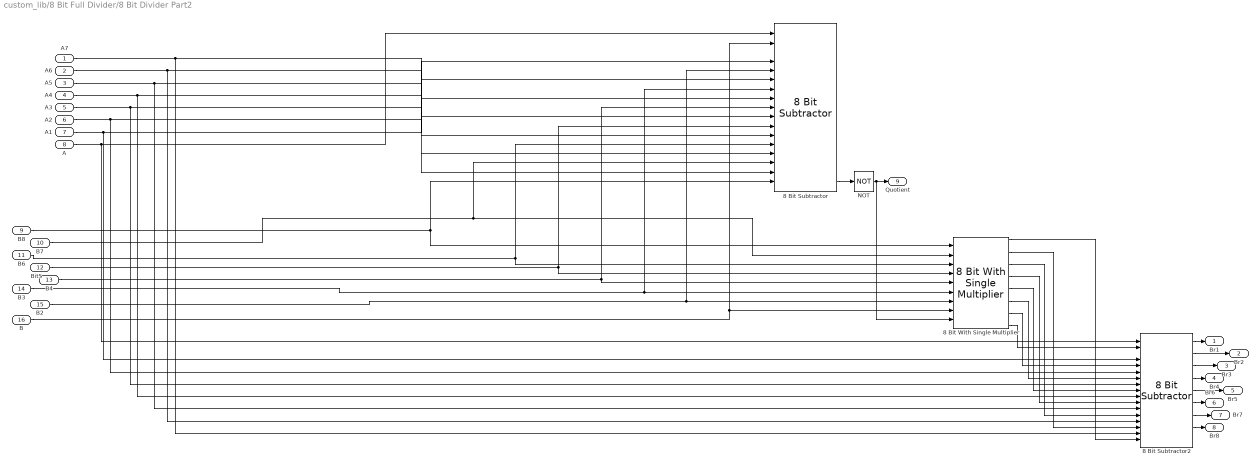
== system custom_lib/8 Bit Full Divider/8 Bit Divider Part2 ==
  A7 : Inport
  A6 : Inport  Port=2
  A5 : Inport  Port=3
  A4 : Inport  Port=4
  A3 : Inport  Port=5
  A2 : Inport  Port=6
  A1 : Inport  Port=7
  A : Inport  Port=8
  B8 : Inport  Port=9
  B7 : Inport  Port=10
  B6 : Inport  Port=11
  Bit5 : Inport  Port=12
  B4 : Inport  Port=13
  B3 : Inport  Port=14
  B2 : Inport  Port=15
  B : Inport  Port=16
  8 Bit Subtractor : $bdroot/8 Bit Subtractor  SystemSampleTime=-1  VariantActivationTime=update diagram  Latency=0  AutoFrameSizeCalculation=off
  8 Bit Subtractor2 : $bdroot/8 Bit Subtractor  SystemSampleTime=-1  VariantActivationTime=update diagram  Latency=0  AutoFrameSizeCalculation=off
  8 Bit With Single Multiplier : $bdroot/8 Bit With Single Multiplier  SystemSampleTime=-1  VariantActivationTime=update diagram  Latency=0  AutoFrameSizeCalculation=off
  NOT : Logic  Operator=NOT  IconShape=distinctive  AllPortsSameDT=off  OutDataTypeStr=boolean
  Br1 : Outport
  Br2 : Outport  Port=2
  Br3 : Outport  Port=3
  Br4 : Outport  Port=4
  Br5 : Outport  Port=5
  Br6 : Outport  Port=6
  Br7 : Outport  Port=7
  Br8 : Outport  Port=8
  Quotient : Outport  Port=9
  wires:
  8 Bit Subtractor2/3 -> Br3/1
  8 Bit With Single Multiplier/2 -> 8 Bit Subtractor2/15
  8 Bit With Single Multiplier/7 -> 8 Bit Subtractor2/5
  B2/1 -> 8 Bit Subtractor/5, 8 Bit With Single Multiplier/7
  B6/1 -> 8 Bit Subtractor/13, 8 Bit With Single Multiplier/3
  8 Bit With Single Multiplier/1 -> 8 Bit Subtractor2/17
  8 Bit Subtractor2/6 -> Br6/1
  A7/1 -> 8 Bit Subtractor2/16, 8 Bit Subtractor/16
  NOT/1 -> Quotient/1, 8 Bit With Single Multiplier/9
  B8/1 -> 8 Bit Subtractor/17, 8 Bit With Single Multiplier/1
  A/1 -> 8 Bit Subtractor2/1, 8 Bit Subtractor/1
  A3/1 -> 8 Bit Subtractor2/8, 8 Bit Subtractor/8
  8 Bit Subtractor2/8 -> Br8/1
  B4/1 -> 8 Bit Subtractor/9, 8 Bit With Single Multiplier/5
  A2/1 -> 8 Bit Subtractor2/6, 8 Bit Subtractor/6
  8 Bit Subtractor2/2 -> Br2/1
  8 Bit With Single Multiplier/3 -> 8 Bit Subtractor2/13
  B7/1 -> 8 Bit With Single Multiplier/2, 8 Bit Subtractor/15
  8 Bit Subtractor/9 -> NOT/1
  B3/1 -> 8 Bit Subtractor/7, 8 Bit With Single Multiplier/6
  Bit5/1 -> 8 Bit Subtractor/11, 8 Bit With Single Multiplier/4
  8 Bit With Single Multiplier/8 -> 8 Bit Subtractor2/2
  8 Bit With Single Multiplier/5 -> 8 Bit Subtractor2/9
  8 Bit With Single Multiplier/6 -> 8 Bit Subtractor2/7
  8 Bit Subtractor2/4 -> Br4/1
  8 Bit Subtractor2/7 -> Br7/1
  8 Bit With Single Multiplier/4 -> 8 Bit Subtractor2/11
  B/1 -> 8 Bit With Single Multiplier/8, 8 Bit Subtractor/2
  8 Bit Subtractor2/5 -> Br5/1
  A1/1 -> 8 Bit Subtractor2/4, 8 Bit Subtractor/4
  A6/1 -> 8 Bit Subtractor2/14, 8 Bit Subtractor/14
  8 Bit Subtractor2/1 -> Br1/1
  A4/1 -> 8 Bit Subtractor2/10, 8 Bit Subtractor/10
  A5/1 -> 8 Bit Subtractor2/12, 8 Bit Subtractor/12

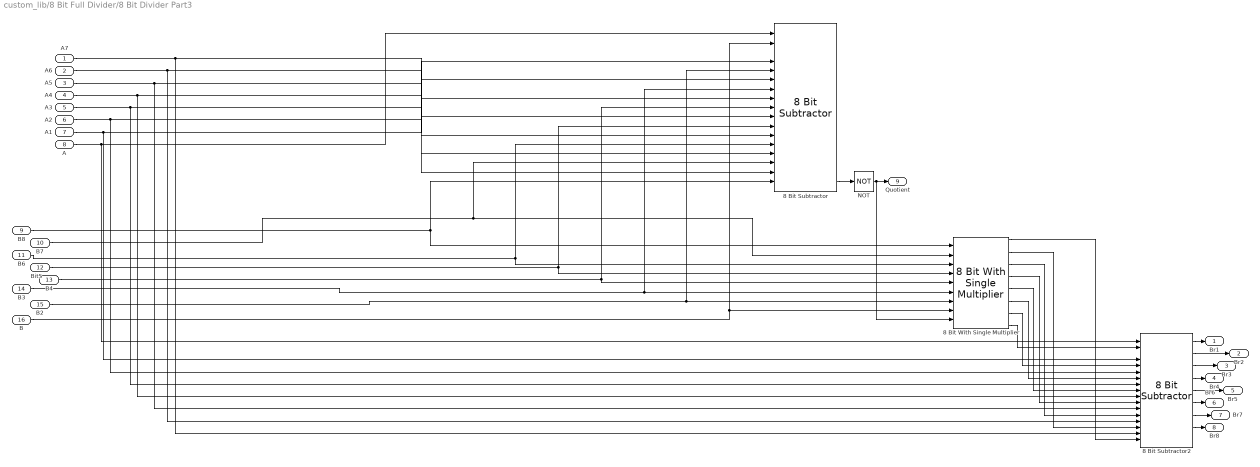
== system custom_lib/8 Bit Full Divider/8 Bit Divider Part3 ==
  A7 : Inport
  A6 : Inport  Port=2
  A5 : Inport  Port=3
  A4 : Inport  Port=4
  A3 : Inport  Port=5
  A2 : Inport  Port=6
  A1 : Inport  Port=7
  A : Inport  Port=8
  B8 : Inport  Port=9
  B7 : Inport  Port=10
  B6 : Inport  Port=11
  Bit5 : Inport  Port=12
  B4 : Inport  Port=13
  B3 : Inport  Port=14
  B2 : Inport  Port=15
  B : Inport  Port=16
  8 Bit Subtractor : $bdroot/8 Bit Subtractor  SystemSampleTime=-1  VariantActivationTime=update diagram  Latency=0  AutoFrameSizeCalculation=off
  8 Bit Subtractor2 : $bdroot/8 Bit Subtractor  SystemSampleTime=-1  VariantActivationTime=update diagram  Latency=0  AutoFrameSizeCalculation=off
  8 Bit With Single Multiplier : $bdroot/8 Bit With Single Multiplier  SystemSampleTime=-1  VariantActivationTime=update diagram  Latency=0  AutoFrameSizeCalculation=off
  NOT : Logic  Operator=NOT  IconShape=distinctive  AllPortsSameDT=off  OutDataTypeStr=boolean
  Br1 : Outport
  Br2 : Outport  Port=2
  Br3 : Outport  Port=3
  Br4 : Outport  Port=4
  Br5 : Outport  Port=5
  Br6 : Outport  Port=6
  Br7 : Outport  Port=7
  Br8 : Outport  Port=8
  Quotient : Outport  Port=9
  wires:
  8 Bit Subtractor2/3 -> Br3/1
  8 Bit With Single Multiplier/2 -> 8 Bit Subtractor2/15
  8 Bit With Single Multiplier/7 -> 8 Bit Subtractor2/5
  B2/1 -> 8 Bit Subtractor/5, 8 Bit With Single Multiplier/7
  B6/1 -> 8 Bit Subtractor/13, 8 Bit With Single Multiplier/3
  8 Bit With Single Multiplier/1 -> 8 Bit Subtractor2/17
  8 Bit Subtractor2/6 -> Br6/1
  A7/1 -> 8 Bit Subtractor2/16, 8 Bit Subtractor/16
  NOT/1 -> Quotient/1, 8 Bit With Single Multiplier/9
  B8/1 -> 8 Bit Subtractor/17, 8 Bit With Single Multiplier/1
  A/1 -> 8 Bit Subtractor2/1, 8 Bit Subtractor/1
  A3/1 -> 8 Bit Subtractor2/8, 8 Bit Subtractor/8
  8 Bit Subtractor2/8 -> Br8/1
  B4/1 -> 8 Bit Subtractor/9, 8 Bit With Single Multiplier/5
  A2/1 -> 8 Bit Subtractor2/6, 8 Bit Subtractor/6
  8 Bit Subtractor2/2 -> Br2/1
  8 Bit With Single Multiplier/3 -> 8 Bit Subtractor2/13
  B7/1 -> 8 Bit With Single Multiplier/2, 8 Bit Subtractor/15
  8 Bit Subtractor/9 -> NOT/1
  B3/1 -> 8 Bit Subtractor/7, 8 Bit With Single Multiplier/6
  Bit5/1 -> 8 Bit Subtractor/11, 8 Bit With Single Multiplier/4
  8 Bit With Single Multiplier/8 -> 8 Bit Subtractor2/2
  8 Bit With Single Multiplier/5 -> 8 Bit Subtractor2/9
  8 Bit With Single Multiplier/6 -> 8 Bit Subtractor2/7
  8 Bit Subtractor2/4 -> Br4/1
  8 Bit Subtractor2/7 -> Br7/1
  8 Bit With Single Multiplier/4 -> 8 Bit Subtractor2/11
  B/1 -> 8 Bit With Single Multiplier/8, 8 Bit Subtractor/2
  8 Bit Subtractor2/5 -> Br5/1
  A1/1 -> 8 Bit Subtractor2/4, 8 Bit Subtractor/4
  A6/1 -> 8 Bit Subtractor2/14, 8 Bit Subtractor/14
  8 Bit Subtractor2/1 -> Br1/1
  A4/1 -> 8 Bit Subtractor2/10, 8 Bit Subtractor/10
  A5/1 -> 8 Bit Subtractor2/12, 8 Bit Subtractor/12

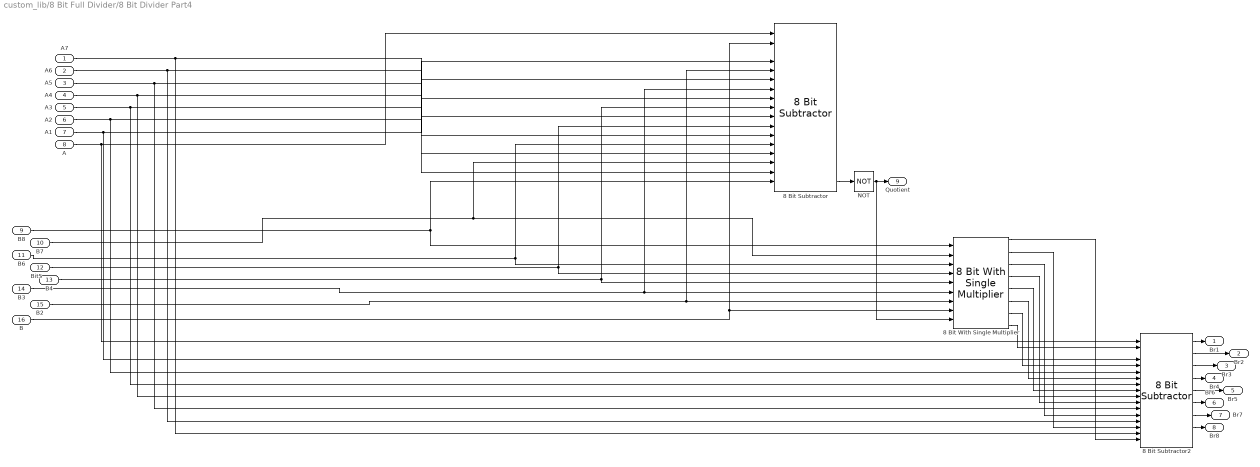
== system custom_lib/8 Bit Full Divider/8 Bit Divider Part4 ==
  A7 : Inport
  A6 : Inport  Port=2
  A5 : Inport  Port=3
  A4 : Inport  Port=4
  A3 : Inport  Port=5
  A2 : Inport  Port=6
  A1 : Inport  Port=7
  A : Inport  Port=8
  B8 : Inport  Port=9
  B7 : Inport  Port=10
  B6 : Inport  Port=11
  Bit5 : Inport  Port=12
  B4 : Inport  Port=13
  B3 : Inport  Port=14
  B2 : Inport  Port=15
  B : Inport  Port=16
  8 Bit Subtractor : $bdroot/8 Bit Subtractor  SystemSampleTime=-1  VariantActivationTime=update diagram  Latency=0  AutoFrameSizeCalculation=off
  8 Bit Subtractor2 : $bdroot/8 Bit Subtractor  SystemSampleTime=-1  VariantActivationTime=update diagram  Latency=0  AutoFrameSizeCalculation=off
  8 Bit With Single Multiplier : $bdroot/8 Bit With Single Multiplier  SystemSampleTime=-1  VariantActivationTime=update diagram  Latency=0  AutoFrameSizeCalculation=off
  NOT : Logic  Operator=NOT  IconShape=distinctive  AllPortsSameDT=off  OutDataTypeStr=boolean
  Br1 : Outport
  Br2 : Outport  Port=2
  Br3 : Outport  Port=3
  Br4 : Outport  Port=4
  Br5 : Outport  Port=5
  Br6 : Outport  Port=6
  Br7 : Outport  Port=7
  Br8 : Outport  Port=8
  Quotient : Outport  Port=9
  wires:
  8 Bit Subtractor2/3 -> Br3/1
  8 Bit With Single Multiplier/2 -> 8 Bit Subtractor2/15
  8 Bit With Single Multiplier/7 -> 8 Bit Subtractor2/5
  B2/1 -> 8 Bit Subtractor/5, 8 Bit With Single Multiplier/7
  B6/1 -> 8 Bit Subtractor/13, 8 Bit With Single Multiplier/3
  8 Bit With Single Multiplier/1 -> 8 Bit Subtractor2/17
  8 Bit Subtractor2/6 -> Br6/1
  A7/1 -> 8 Bit Subtractor2/16, 8 Bit Subtractor/16
  NOT/1 -> Quotient/1, 8 Bit With Single Multiplier/9
  B8/1 -> 8 Bit Subtractor/17, 8 Bit With Single Multiplier/1
  A/1 -> 8 Bit Subtractor2/1, 8 Bit Subtractor/1
  A3/1 -> 8 Bit Subtractor2/8, 8 Bit Subtractor/8
  8 Bit Subtractor2/8 -> Br8/1
  B4/1 -> 8 Bit Subtractor/9, 8 Bit With Single Multiplier/5
  A2/1 -> 8 Bit Subtractor2/6, 8 Bit Subtractor/6
  8 Bit Subtractor2/2 -> Br2/1
  8 Bit With Single Multiplier/3 -> 8 Bit Subtractor2/13
  B7/1 -> 8 Bit With Single Multiplier/2, 8 Bit Subtractor/15
  8 Bit Subtractor/9 -> NOT/1
  B3/1 -> 8 Bit Subtractor/7, 8 Bit With Single Multiplier/6
  Bit5/1 -> 8 Bit Subtractor/11, 8 Bit With Single Multiplier/4
  8 Bit With Single Multiplier/8 -> 8 Bit Subtractor2/2
  8 Bit With Single Multiplier/5 -> 8 Bit Subtractor2/9
  8 Bit With Single Multiplier/6 -> 8 Bit Subtractor2/7
  8 Bit Subtractor2/4 -> Br4/1
  8 Bit Subtractor2/7 -> Br7/1
  8 Bit With Single Multiplier/4 -> 8 Bit Subtractor2/11
  B/1 -> 8 Bit With Single Multiplier/8, 8 Bit Subtractor/2
  8 Bit Subtractor2/5 -> Br5/1
  A1/1 -> 8 Bit Subtractor2/4, 8 Bit Subtractor/4
  A6/1 -> 8 Bit Subtractor2/14, 8 Bit Subtractor/14
  8 Bit Subtractor2/1 -> Br1/1
  A4/1 -> 8 Bit Subtractor2/10, 8 Bit Subtractor/10
  A5/1 -> 8 Bit Subtractor2/12, 8 Bit Subtractor/12

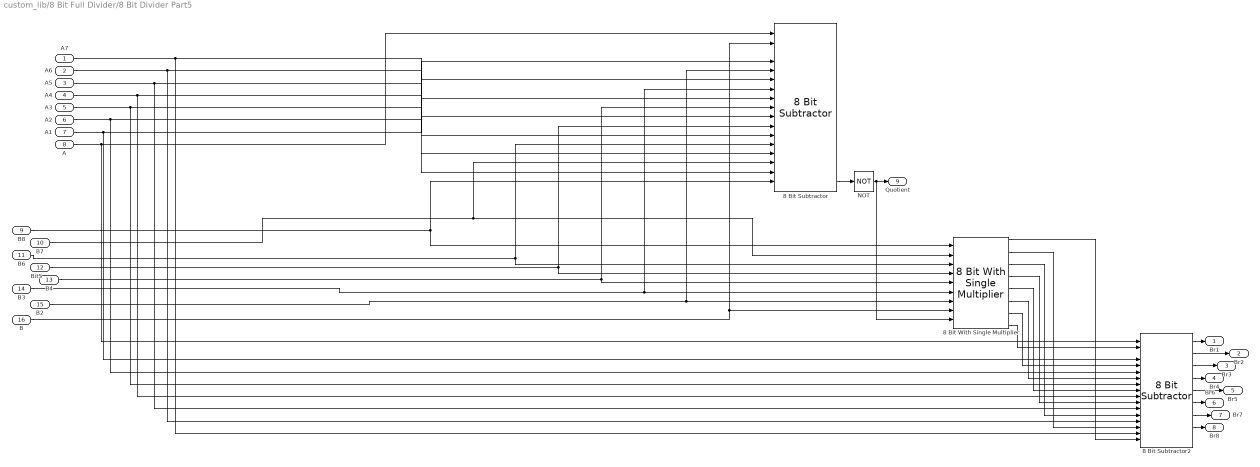
== system custom_lib/8 Bit Full Divider/8 Bit Divider Part5 ==
  A7 : Inport
  A6 : Inport  Port=2
  A5 : Inport  Port=3
  A4 : Inport  Port=4
  A3 : Inport  Port=5
  A2 : Inport  Port=6
  A1 : Inport  Port=7
  A : Inport  Port=8
  B8 : Inport  Port=9
  B7 : Inport  Port=10
  B6 : Inport  Port=11
  Bit5 : Inport  Port=12
  B4 : Inport  Port=13
  B3 : Inport  Port=14
  B2 : Inport  Port=15
  B : Inport  Port=16
  8 Bit Subtractor : $bdroot/8 Bit Subtractor  SystemSampleTime=-1  VariantActivationTime=update diagram  Latency=0  AutoFrameSizeCalculation=off
  8 Bit Subtractor2 : $bdroot/8 Bit Subtractor  SystemSampleTime=-1  VariantActivationTime=update diagram  Latency=0  AutoFrameSizeCalculation=off
  8 Bit With Single Multiplier : $bdroot/8 Bit With Single Multiplier  SystemSampleTime=-1  VariantActivationTime=update diagram  Latency=0  AutoFrameSizeCalculation=off
  NOT : Logic  Operator=NOT  IconShape=distinctive  AllPortsSameDT=off  OutDataTypeStr=boolean
  Br1 : Outport
  Br2 : Outport  Port=2
  Br3 : Outport  Port=3
  Br4 : Outport  Port=4
  Br5 : Outport  Port=5
  Br6 : Outport  Port=6
  Br7 : Outport  Port=7
  Br8 : Outport  Port=8
  Quotient : Outport  Port=9
  wires:
  8 Bit Subtractor2/3 -> Br3/1
  8 Bit With Single Multiplier/2 -> 8 Bit Subtractor2/15
  8 Bit With Single Multiplier/7 -> 8 Bit Subtractor2/5
  B2/1 -> 8 Bit Subtractor/5, 8 Bit With Single Multiplier/7
  B6/1 -> 8 Bit Subtractor/13, 8 Bit With Single Multiplier/3
  8 Bit With Single Multiplier/1 -> 8 Bit Subtractor2/17
  8 Bit Subtractor2/6 -> Br6/1
  A7/1 -> 8 Bit Subtractor2/16, 8 Bit Subtractor/16
  NOT/1 -> Quotient/1, 8 Bit With Single Multiplier/9
  B8/1 -> 8 Bit Subtractor/17, 8 Bit With Single Multiplier/1
  A/1 -> 8 Bit Subtractor2/1, 8 Bit Subtractor/1
  A3/1 -> 8 Bit Subtractor2/8, 8 Bit Subtractor/8
  8 Bit Subtractor2/8 -> Br8/1
  B4/1 -> 8 Bit Subtractor/9, 8 Bit With Single Multiplier/5
  A2/1 -> 8 Bit Subtractor2/6, 8 Bit Subtractor/6
  8 Bit Subtractor2/2 -> Br2/1
  8 Bit With Single Multiplier/3 -> 8 Bit Subtractor2/13
  B7/1 -> 8 Bit With Single Multiplier/2, 8 Bit Subtractor/15
  8 Bit Subtractor/9 -> NOT/1
  B3/1 -> 8 Bit Subtractor/7, 8 Bit With Single Multiplier/6
  Bit5/1 -> 8 Bit Subtractor/11, 8 Bit With Single Multiplier/4
  8 Bit With Single Multiplier/8 -> 8 Bit Subtractor2/2
  8 Bit With Single Multiplier/5 -> 8 Bit Subtractor2/9
  8 Bit With Single Multiplier/6 -> 8 Bit Subtractor2/7
  8 Bit Subtractor2/4 -> Br4/1
  8 Bit Subtractor2/7 -> Br7/1
  8 Bit With Single Multiplier/4 -> 8 Bit Subtractor2/11
  B/1 -> 8 Bit With Single Multiplier/8, 8 Bit Subtractor/2
  8 Bit Subtractor2/5 -> Br5/1
  A1/1 -> 8 Bit Subtractor2/4, 8 Bit Subtractor/4
  A6/1 -> 8 Bit Subtractor2/14, 8 Bit Subtractor/14
  8 Bit Subtractor2/1 -> Br1/1
  A4/1 -> 8 Bit Subtractor2/10, 8 Bit Subtractor/10
  A5/1 -> 8 Bit Subtractor2/12, 8 Bit Subtractor/12

== system custom_lib/8 Bit Full Divider/8 Bit Divider Part6 ==
  A7 : Inport
  A6 : Inport  Port=2
  A5 : Inport  Port=3
  A4 : Inport  Port=4
  A3 : Inport  Port=5
  A2 : Inport  Port=6
  A1 : Inport  Port=7
  A : Inport  Port=8
  B8 : Inport  Port=9
  B7 : Inport  Port=10
  B6 : Inport  Port=11
  Bit5 : Inport  Port=12
  B4 : Inport  Port=13
  B3 : Inport  Port=14
  B2 : Inport  Port=15
  B : Inport  Port=16
  8 Bit Subtractor : $bdroot/8 Bit Subtractor  SystemSampleTime=-1  VariantActivationTime=update diagram  Latency=0  AutoFrameSizeCalculation=off
  8 Bit Subtractor2 : $bdroot/8 Bit Subtractor  SystemSampleTime=-1  VariantActivationTime=update diagram  Latency=0  AutoFrameSizeCalculation=off
  8 Bit With Single Multiplier : $bdroot/8 Bit With Single Multiplier  SystemSampleTime=-1  VariantActivationTime=update diagram  Latency=0  AutoFrameSizeCalculation=off
  NOT : Logic  Operator=NOT  IconShape=distinctive  AllPortsSameDT=off  OutDataTypeStr=boolean
  Br1 : Outport
  Br2 : Outport  Port=2
  Br3 : Outport  Port=3
  Br4 : Outport  Port=4
  Br5 : Outport  Port=5
  Br6 : Outport  Port=6
  Br7 : Outport  Port=7
  Br8 : Outport  Port=8
  Quotient : Outport  Port=9
  wires:
  8 Bit Subtractor2/3 -> Br3/1
  8 Bit With Single Multiplier/2 -> 8 Bit Subtractor2/15
  8 Bit With Single Multiplier/7 -> 8 Bit Subtractor2/5
  B2/1 -> 8 Bit Subtractor/5, 8 Bit With Single Multiplier/7
  B6/1 -> 8 Bit Subtractor/13, 8 Bit With Single Multiplier/3
  8 Bit With Single Multiplier/1 -> 8 Bit Subtractor2/17
  8 Bit Subtractor2/6 -> Br6/1
  A7/1 -> 8 Bit Subtractor2/16, 8 Bit Subtractor/16
  NOT/1 -> Quotient/1, 8 Bit With Single Multiplier/9
  B8/1 -> 8 Bit Subtractor/17, 8 Bit With Single Multiplier/1
  A/1 -> 8 Bit Subtractor2/1, 8 Bit Subtractor/1
  A3/1 -> 8 Bit Subtractor2/8, 8 Bit Subtractor/8
  8 Bit Subtractor2/8 -> Br8/1
  B4/1 -> 8 Bit Subtractor/9, 8 Bit With Single Multiplier/5
  A2/1 -> 8 Bit Subtractor2/6, 8 Bit Subtractor/6
  8 Bit Subtractor2/2 -> Br2/1
  8 Bit With Single Multiplier/3 -> 8 Bit Subtractor2/13
  B7/1 -> 8 Bit With Single Multiplier/2, 8 Bit Subtractor/15
  8 Bit Subtractor/9 -> NOT/1
  B3/1 -> 8 Bit Subtractor/7, 8 Bit With Single Multiplier/6
  Bit5/1 -> 8 Bit Subtractor/11, 8 Bit With Single Multiplier/4
  8 Bit With Single Multiplier/8 -> 8 Bit Subtractor2/2
  8 Bit With Single Multiplier/5 -> 8 Bit Subtractor2/9
  8 Bit With Single Multiplier/6 -> 8 Bit Subtractor2/7
  8 Bit Subtractor2/4 -> Br4/1
  8 Bit Subtractor2/7 -> Br7/1
  8 Bit With Single Multiplier/4 -> 8 Bit Subtractor2/11
  B/1 -> 8 Bit With Single Multiplier/8, 8 Bit Subtractor/2
  8 Bit Subtractor2/5 -> Br5/1
  A1/1 -> 8 Bit Subtractor2/4, 8 Bit Subtractor/4
  A6/1 -> 8 Bit Subtractor2/14, 8 Bit Subtractor/14
  8 Bit Subtractor2/1 -> Br1/1
  A4/1 -> 8 Bit Subtractor2/10, 8 Bit Subtractor/10
  A5/1 -> 8 Bit Subtractor2/12, 8 Bit Subtractor/12

== system custom_lib/8 Bit Full Divider/8 Bit Divider Part7 ==
  A7 : Inport
  A6 : Inport  Port=2
  A5 : Inport  Port=3
  A4 : Inport  Port=4
  A3 : Inport  Port=5
  A2 : Inport  Port=6
  A1 : Inport  Port=7
  A : Inport  Port=8
  B8 : Inport  Port=9
  B7 : Inport  Port=10
  B6 : Inport  Port=11
  Bit5 : Inport  Port=12
  B4 : Inport  Port=13
  B3 : Inport  Port=14
  B2 : Inport  Port=15
  B : Inport  Port=16
  8 Bit Subtractor : $bdroot/8 Bit Subtractor  SystemSampleTime=-1  VariantActivationTime=update diagram  Latency=0  AutoFrameSizeCalculation=off
  8 Bit Subtractor2 : $bdroot/8 Bit Subtractor  SystemSampleTime=-1  VariantActivationTime=update diagram  Latency=0  AutoFrameSizeCalculation=off
  8 Bit With Single Multiplier : $bdroot/8 Bit With Single Multiplier  SystemSampleTime=-1  VariantActivationTime=update diagram  Latency=0  AutoFrameSizeCalculation=off
  NOT : Logic  Operator=NOT  IconShape=distinctive  AllPortsSameDT=off  OutDataTypeStr=boolean
  Br1 : Outport
  Br2 : Outport  Port=2
  Br3 : Outport  Port=3
  Br4 : Outport  Port=4
  Br5 : Outport  Port=5
  Br6 : Outport  Port=6
  Br7 : Outport  Port=7
  Br8 : Outport  Port=8
  Quotient : Outport  Port=9
  wires:
  8 Bit Subtractor2/3 -> Br3/1
  8 Bit With Single Multiplier/2 -> 8 Bit Subtractor2/15
  8 Bit With Single Multiplier/7 -> 8 Bit Subtractor2/5
  B2/1 -> 8 Bit Subtractor/5, 8 Bit With Single Multiplier/7
  B6/1 -> 8 Bit Subtractor/13, 8 Bit With Single Multiplier/3
  8 Bit With Single Multiplier/1 -> 8 Bit Subtractor2/17
  8 Bit Subtractor2/6 -> Br6/1
  A7/1 -> 8 Bit Subtractor2/16, 8 Bit Subtractor/16
  NOT/1 -> Quotient/1, 8 Bit With Single Multiplier/9
  B8/1 -> 8 Bit Subtractor/17, 8 Bit With Single Multiplier/1
  A/1 -> 8 Bit Subtractor2/1, 8 Bit Subtractor/1
  A3/1 -> 8 Bit Subtractor2/8, 8 Bit Subtractor/8
  8 Bit Subtractor2/8 -> Br8/1
  B4/1 -> 8 Bit Subtractor/9, 8 Bit With Single Multiplier/5
  A2/1 -> 8 Bit Subtractor2/6, 8 Bit Subtractor/6
  8 Bit Subtractor2/2 -> Br2/1
  8 Bit With Single Multiplier/3 -> 8 Bit Subtractor2/13
  B7/1 -> 8 Bit With Single Multiplier/2, 8 Bit Subtractor/15
  8 Bit Subtractor/9 -> NOT/1
  B3/1 -> 8 Bit Subtractor/7, 8 Bit With Single Multiplier/6
  Bit5/1 -> 8 Bit Subtractor/11, 8 Bit With Single Multiplier/4
  8 Bit With Single Multiplier/8 -> 8 Bit Subtractor2/2
  8 Bit With Single Multiplier/5 -> 8 Bit Subtractor2/9
  8 Bit With Single Multiplier/6 -> 8 Bit Subtractor2/7
  8 Bit Subtractor2/4 -> Br4/1
  8 Bit Subtractor2/7 -> Br7/1
  8 Bit With Single Multiplier/4 -> 8 Bit Subtractor2/11
  B/1 -> 8 Bit With Single Multiplier/8, 8 Bit Subtractor/2
  8 Bit Subtractor2/5 -> Br5/1
  A1/1 -> 8 Bit Subtractor2/4, 8 Bit Subtractor/4
  A6/1 -> 8 Bit Subtractor2/14, 8 Bit Subtractor/14
  8 Bit Subtractor2/1 -> Br1/1
  A4/1 -> 8 Bit Subtractor2/10, 8 Bit Subtractor/10
  A5/1 -> 8 Bit Subtractor2/12, 8 Bit Subtractor/12

== matlab function custom_lib/Binary To Decimal ==
  data: decimal output; bit8 input; bit7 input; bit6 input; bit5 input; bit4 input; bit3 input; bit2 input; bit1 input
function decimal = fcn(bit8, bit7, bit6, bit5, bit4, bit3, bit2, bit1)

decimal = (bit1 * 2^0) + (bit2 * 2^1) + (bit3 * 2^2) + (bit4 * 2^3) + (bit5 * 2^4) + (bit6 * 2^5) + (bit7 * 2^6) + (bit8 * 2^7);

== matlab function custom_lib/Decimal To Binary ==
  data: decimal input; bit8 output; bit7 output; bit6 output; bit5 output; bit4 output; bit3 output; bit2 output; bit1 output
function [bit8, bit7, bit6, bit5, bit4, bit3, bit2, bit1] = fcn(decimal)

bits = [0,0,0,0,0,0,0,0];

counter = 1;
while(counter<=8)
    bits(counter) = floor(mod(decimal,2));
    decimal=decimal/2;
    counter=counter+1;
end


bit1 = bits(1);
bit2 = bits(2);
bit3 = bits(3);
bit4 = bits(4);
bit5 = bits(5);
bit6 = bits(6);
bit7 = bits(7);
bit8 = bits(8);

== matlab function custom_lib/8 Bit Decimal Parts Divider ==
  data: decimal input; hundreds output; tens output; ones output
function [hundreds,tens, ones] = fcn(decimal)

hundreds = floor(decimal / 100);
tens = floor((mod(decimal,100))/10);
ones = floor(mod(decimal,10));
